simulink model "torpedo"  (Simulink 7.6)
settings: Solver=FixedStepDiscrete  StartTime=0.0  StopTime=0  FixedStep=1/30  RelTol=1e-3
values from neighbouring files (symbols this model uses):
  Forward_Camera_Dimensions = [640 480]    [VisionConstants.m]
  Iter_Segment_Thresh = 60    [VisionConstants.m]
undefined symbols (not defined in the file or in its folder): a_range, b_range, eccent_range, extent_range, Rec, SDTV
libraries: vipgeotforms x3, vipconversions x1
settings Model: Creator=auvt  LastModifiedBy=auvt
settings RTWCC: TargetLang=C++

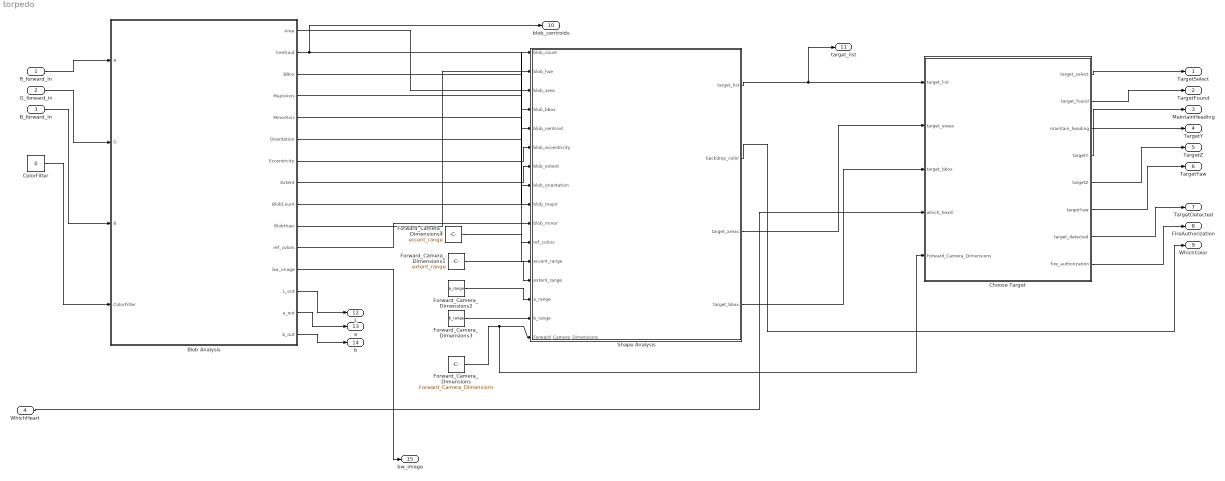
== system torpedo ==
  R_forward_in : Inport  PortDimensions=Forward_Camera_Dimensions
  G_forward_in : Inport  Port=2  PortDimensions=Forward_Camera_Dimensions
  B_forward_in : Inport  Port=3  PortDimensions=Forward_Camera_Dimensions
  WhichHeart : Inport  Port=4
  Blob Analysis : Subsystem
  Choose Target : Stateflow chart  TreatAsAtomicUnit=on
  ColorFilter : Constant  Value=0  SampleTime=-1
  Forward_Camera_Dimensions : Constant  Value=Forward_Camera_Dimensions  SampleTime=-1
  Forward_Camera_Dimensions1 : Constant  Value=extent_range  SampleTime=-1
  Forward_Camera_Dimensions2 : Constant  Value=a_range  SampleTime=-1
  Forward_Camera_Dimensions3 : Constant  Value=b_range  SampleTime=-1
  Forward_Camera_Dimensions4 : Constant  Value=eccent_range  SampleTime=-1
  Shape Analysis : Stateflow chart  TreatAsAtomicUnit=on
  TargetSelect : Outport  OutDataTypeStr=double
  TargetFound : Outport  Port=2  OutDataTypeStr=double
  MaintainHeading : Outport  Port=3  OutDataTypeStr=double
  TargetY : Outport  Port=4  OutDataTypeStr=double
  TargetZ : Outport  Port=5  OutDataTypeStr=double
  TargetYaw : Outport  Port=6  OutDataTypeStr=double
  TargetDetected : Outport  Port=7  OutDataTypeStr=double
  FireAuthorization : Outport  Port=8  OutDataTypeStr=double
  WhichColor : Outport  Port=9  OutDataTypeStr=double
  blob_centroids : Outport  Port=10  OutDataTypeStr=double
  target_list : Outport  Port=11  OutDataTypeStr=double
  L : Outport  Port=12
  a : Outport  Port=13
  b : Outport  Port=14
  bw_image : Outport  Port=15  OutDataTypeStr=double
  wires:
  Shape Analysis/2(backdrop_color) -> WhichColor/1
  Shape Analysis/1(target_list) -> Choose Target/1(target_list), target_list/1
  WhichHeart/1 -> Choose Target/4(which_heart)
  Choose Target/1(target_select) -> TargetSelect/1
  Choose Target/2(target_found) -> TargetFound/1
  Choose Target/3(maintain_heading) -> MaintainHeading/1
  Choose Target/4(targetY) -> TargetY/1
  Choose Target/5(targetZ) -> TargetZ/1
  Choose Target/6(targetYaw) -> TargetYaw/1
  Choose Target/7(target_detected) -> TargetDetected/1
  Choose Target/8(fire_authorization) -> FireAuthorization/1
  Shape Analysis/3(target_areas) -> Choose Target/2(target_areas)
  Shape Analysis/4(target_bbox) -> Choose Target/3(target_bbox)
  Forward_Camera_Dimensions/1 -> Shape Analysis/16(Forward_Camera_Dimensions), Choose Target/5(Forward_Camera_Dimensions)
  Forward_Camera_Dimensions3/1 -> Shape Analysis/15(b_range)
  Forward_Camera_Dimensions2/1 -> Shape Analysis/14(a_range)
  Forward_Camera_Dimensions1/1 -> Shape Analysis/13(extent_range)
  Forward_Camera_Dimensions4/1 -> Shape Analysis/12(eccent_range)
  R_forward_in/1 -> Blob Analysis/1(R)
  G_forward_in/1 -> Blob Analysis/2(G)
  B_forward_in/1 -> Blob Analysis/3(B)
  ColorFilter/1 -> Blob Analysis/4(ColorFilter)
  Blob Analysis/1(Area) -> Shape Analysis/3(blob_area)
  Blob Analysis/9(BlobCount) -> Shape Analysis/1(blob_count)
  Blob Analysis/10(BlobHues) -> Shape Analysis/2(blob_hue)
  Blob Analysis/3(BBox) -> Shape Analysis/4(blob_bbox)
  Blob Analysis/2(Centroid) -> Shape Analysis/5(blob_centroid), blob_centroids/1
  Blob Analysis/7(Eccentricity) -> Shape Analysis/6(blob_eccentricity)
  Blob Analysis/8(Extent) -> Shape Analysis/7(blob_extent)
  Blob Analysis/6(Orientation) -> Shape Analysis/8(blob_orientation)
  Blob Analysis/4(MajorAxis) -> Shape Analysis/9(blob_major)
  Blob Analysis/5(MinorAxis) -> Shape Analysis/10(blob_minor)
  Blob Analysis/11(ref_colors) -> Shape Analysis/11(ref_colors)
  Blob Analysis/13(L_out) -> L/1
  Blob Analysis/14(a_out) -> a/1
  Blob Analysis/15(b_out) -> b/1
  Blob Analysis/12(bw_image) -> bw_image/1

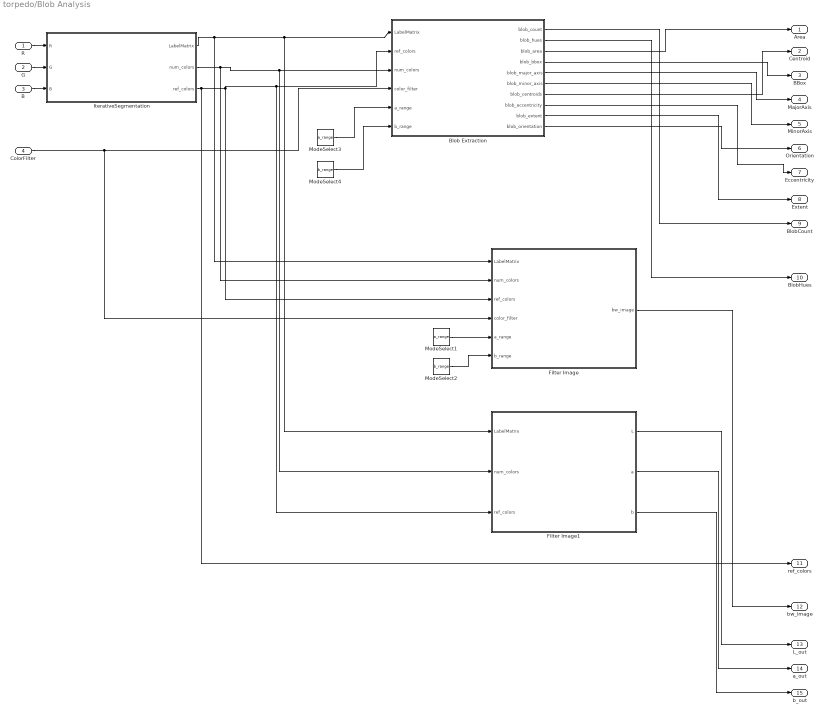
== system torpedo/Blob Analysis ==
  R : Inport
  G : Inport  Port=2
  B : Inport  Port=3
  ColorFilter : Inport  Port=4
  Blob Extraction : Stateflow chart  TreatAsAtomicUnit=on
  Filter Image : Stateflow chart  TreatAsAtomicUnit=on
  Filter Image1 : Stateflow chart  TreatAsAtomicUnit=on
  IterativeSegmentation : Subsystem
      settings: UndoDeleteFcn=Stateflow.SLINSF.SimulinkMan.restorePreDeleteFcn  PreDeleteFcn=Stateflow.SLINSF.SimulinkMan.removePreDeleteFcn
  ModeSelect1 : Constant  Value=a_range  SampleTime=-1
  ModeSelect2 : Constant  Value=b_range  SampleTime=-1
  ModeSelect3 : Constant  Value=a_range  SampleTime=-1
  ModeSelect4 : Constant  Value=b_range  SampleTime=-1
  Area : Outport
  Centroid : Outport  Port=2
  BBox : Outport  Port=3
  MajorAxis : Outport  Port=4
  MinorAxis : Outport  Port=5
  Orientation : Outport  Port=6
  Eccentricity : Outport  Port=7
  Extent : Outport  Port=8
  BlobCount : Outport  Port=9
  BlobHues : Outport  Port=10
  ref_colors : Outport  Port=11
  bw_image : Outport  Port=12
  L_out : Outport  Port=13
  a_out : Outport  Port=14
  b_out : Outport  Port=15
  wires:
  R/1 -> IterativeSegmentation/1(R)
  G/1 -> IterativeSegmentation/2(G)
  B/1 -> IterativeSegmentation/3(B)
  IterativeSegmentation/1(LabelMatrix) -> Filter Image/1(LabelMatrix), Blob Extraction/1(LabelMatrix), Filter Image1/1(LabelMatrix)
  IterativeSegmentation/2(num_colors) -> Filter Image/2(num_colors), Blob Extraction/3(num_colors), Filter Image1/2(num_colors)
  IterativeSegmentation/3(ref_colors) -> Filter Image/3(ref_colors), Blob Extraction/2(ref_colors), Filter Image1/3(ref_colors), ref_colors/1
  ModeSelect1/1 -> Filter Image/5(a_range)
  ModeSelect2/1 -> Filter Image/6(b_range)
  ModeSelect3/1 -> Blob Extraction/5(a_range)
  ModeSelect4/1 -> Blob Extraction/6(b_range)
  ColorFilter/1 -> Blob Extraction/4(color_filter), Filter Image/4(color_filter)
  Blob Extraction/3(blob_area) -> Area/1
  Blob Extraction/7(blob_centroids) -> Centroid/1
  Blob Extraction/4(blob_bbox) -> BBox/1
  Blob Extraction/5(blob_major_axis) -> MajorAxis/1
  Blob Extraction/6(blob_minor_axis) -> MinorAxis/1
  Blob Extraction/10(blob_orientation) -> Orientation/1
  Blob Extraction/8(blob_eccentricity) -> Eccentricity/1
  Blob Extraction/9(blob_extent) -> Extent/1
  Blob Extraction/1(blob_count) -> BlobCount/1
  Blob Extraction/2(blob_hues) -> BlobHues/1
  Filter Image/1(bw_image) -> bw_image/1
  Filter Image1/1(L) -> L_out/1
  Filter Image1/2(a) -> a_out/1
  Filter Image1/3(b) -> b_out/1

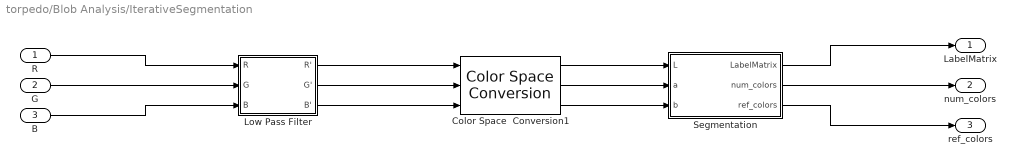
== system torpedo/Blob Analysis/IterativeSegmentation ==
  R : Inport
  G : Inport  Port=2
  B : Inport  Port=3
  Color Space  Conversion1 : vipconversions/Color Space  Conversion  conversion=Obsolete  conversionActive=sR'G'B' to L*a*b*  wp_str=D50  rec=Rec. 601 (SDTV)  sys=1125/60/2:1  imagePorts=Separate color signals
  Low Pass Filter : Subsystem
  Segmentation : Subsystem
  LabelMatrix : Outport
  num_colors : Outport  Port=2
  ref_colors : Outport  Port=3
  wires:
  Segmentation/3(ref_colors) -> ref_colors/1
  Segmentation/2(num_colors) -> num_colors/1
  Segmentation/1(LabelMatrix) -> LabelMatrix/1
  Low Pass Filter/3(B') -> Color Space  Conversion1/3
  Low Pass Filter/2(G') -> Color Space  Conversion1/2
  Low Pass Filter/1(R') -> Color Space  Conversion1/1
  Color Space  Conversion1/3 -> Segmentation/3(b)
  Color Space  Conversion1/2 -> Segmentation/2(a)
  Color Space  Conversion1/1 -> Segmentation/1(L)
  R/1 -> Low Pass Filter/1(R)
  G/1 -> Low Pass Filter/2(G)
  B/1 -> Low Pass Filter/3(B)

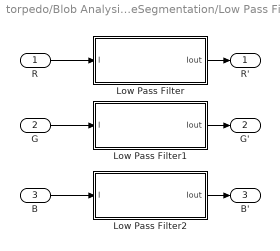
== system torpedo/Blob Analysis/IterativeSegmentation/Low Pass Filter ==
  R : Inport
  G : Inport  Port=2
  B : Inport  Port=3
  Low Pass Filter : Stateflow chart  TreatAsAtomicUnit=on
  Low Pass Filter1 : Stateflow chart  TreatAsAtomicUnit=on
  Low Pass Filter2 : Stateflow chart  TreatAsAtomicUnit=on
  R' : Outport
  G' : Outport  Port=2
  B' : Outport  Port=3
  wires:
  Low Pass Filter/1(Iout) -> R'/1
  Low Pass Filter2/1(Iout) -> B'/1
  Low Pass Filter1/1(Iout) -> G'/1
  B/1 -> Low Pass Filter2/1(I)
  G/1 -> Low Pass Filter1/1(I)
  R/1 -> Low Pass Filter/1(I)

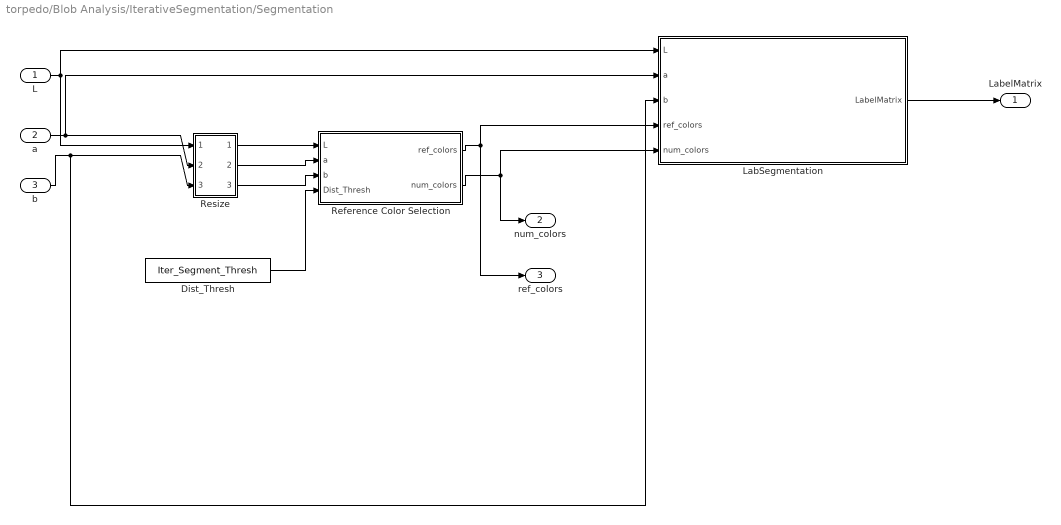
== system torpedo/Blob Analysis/IterativeSegmentation/Segmentation ==
  L : Inport
  a : Inport  Port=2
  b : Inport  Port=3
  Dist_Thresh : Constant  Value=Iter_Segment_Thresh  SampleTime=-1
  LabSegmentation : Stateflow chart  TreatAsAtomicUnit=on
  Reference Color Selection : Stateflow chart  TreatAsAtomicUnit=on
  Resize : Subsystem
  LabelMatrix : Outport
  num_colors : Outport  Port=2
  ref_colors : Outport  Port=3
  wires:
  Dist_Thresh/1 -> Reference Color Selection/4(Dist_Thresh)
  LabSegmentation/1(LabelMatrix) -> LabelMatrix/1
  Reference Color Selection/2(num_colors) -> LabSegmentation/5(num_colors), num_colors/1
  Reference Color Selection/1(ref_colors) -> ref_colors/1, LabSegmentation/4(ref_colors)
  Resize/3(Out3) -> Reference Color Selection/3(b)
  Resize/2(Out2) -> Reference Color Selection/2(a)
  Resize/1(Out1) -> Reference Color Selection/1(L)
  b/1 -> LabSegmentation/3(b), Resize/3(In3)
  a/1 -> LabSegmentation/2(a), Resize/2(In2)
  L/1 -> LabSegmentation/1(L), Resize/1(In1)

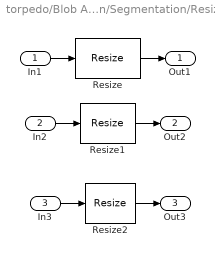
== system torpedo/Blob Analysis/IterativeSegmentation/Segmentation/Resize ==
  In1 : Inport
  In2 : Inport  Port=2
  In3 : Inport  Port=3
  Resize : vipgeotforms/Resize  DialogController=vipDDGCreate  DialogControllerArgs=DataTag0  specify=Number of output rows and columns  rfactor=[]  outCols=25  outRows=25  outRowsCols=[60 80]  interp_method=Bilinear  antialias=on  useROI=off  roiFlag=off  prodOutputMode=Binary point scaling  prodOutputWordLength=32  prodOutputFracLength=10  roundingMode=Nearest  overflowMode=on
  Resize1 : vipgeotforms/Resize  DialogController=vipDDGCreate  DialogControllerArgs=DataTag1  specify=Number of output rows and columns  rfactor=[200 150]  outCols=25  outRows=25  outRowsCols=[60 80]  interp_method=Bilinear  antialias=on  useROI=off  roiFlag=off  prodOutputMode=Binary point scaling  prodOutputWordLength=32  prodOutputFracLength=10  roundingMode=Nearest  overflowMode=on
  Resize2 : vipgeotforms/Resize  DialogController=vipDDGCreate  DialogControllerArgs=DataTag2  specify=Number of output rows and columns  rfactor=[200 150]  outCols=25  outRows=25  outRowsCols=[60 80]  interp_method=Bilinear  antialias=on  useROI=off  roiFlag=off  prodOutputMode=Binary point scaling  prodOutputWordLength=32  prodOutputFracLength=10  roundingMode=Nearest  overflowMode=on
  Out1 : Outport
  Out2 : Outport  Port=2
  Out3 : Outport  Port=3
  wires:
  Resize2/1 -> Out3/1
  In3/1 -> Resize2/1
  Resize1/1 -> Out2/1
  In2/1 -> Resize1/1
  Resize/1 -> Out1/1
  In1/1 -> Resize/1

== matlab function Blob Analysis/Blob Extraction ==
  data: LabelMatrix input double; ref_colors input double; num_colors input double; color_filter input double; blob_count output double; blob_hues output double; blob_area output double; blob_bbox output double; blob_major_axis output double; blob_minor_axis output double; blob_centroids output double; blob_eccentricity output double; blob_extent output double; blob_orientation output double; a_range input double; b_range input double
function [blob_count, blob_hues, blob_area, blob_bbox, blob_major_axis, blob_minor_axis, blob_centroids, blob_eccentricity, blob_extent, blob_orientation] = GetBlobInfo(LabelMatrix, ref_colors, num_colors, color_filter, a_range, b_range)

% This function extracts 
% Input
%   

% Initialize
max_num_blobs = 50;
min_blob_area = 5;

[rows, cols] = size(LabelMatrix);
LogicMatrix = false(rows,cols);

blob_count = 0;
blob_hues = zeros(3,max_num_blobs);

blob_area = -1.*ones(1,max_num_blobs);
blob_bbox = zeros(4,max_num_blobs);
blob_major_axis = zeros(1,max_num_blobs);
blob_minor_axis = zeros(1,max_num_blobs);
blob_centroids = zeros(2,max_num_blobs);
blob_eccentricity = zeros(1,max_num_blobs);
blob_extent = zeros(1,max_num_blobs);
blob_orientation = zeros(1,max_num_blobs);


% Input hblob, a matrix containing [Area, blob_centroids, Eccentricity] for each
% identified blob
persistent hblob
if isempty(hblob)
    hblob = video.BlobAnalysis('AreaOutputPort',true,'CentroidOutputPort',true,...
        'BoundingBoxOutputPort',true,'MajorAxisLengthOutputPort',true,'MinorAxisLengthOutputPort',true,...
        'OrientationOutputPort',true,...
        'EccentricityOutputPort',true,'ExtentOutputPort',true,'NumBlobsOutputPort',true,...
        'MinimumBlobAreaSource','Property','MinimumBlobArea', min_blob_area);
end


% Calculate geometric information about the blobs
%
% LogicMatrix is a binary version of LabelMatrix, with ones at all
%   locations for which color values are k, and zeros everywhere else
for k = 1:num_colors

    a = ref_colors(k, 2);
    b = ref_colors(k, 3);

    if( color_filter == 0 )
        condition = 1;
    else
        if( a >= a_range(1,5) && a <= a_range(2,5) && b >= b_range(1,5) && b <= b_range(2,5) )
            condition = 1;
        else
            condition = 0;
        end
    end
    
    if( condition == 1 )
        
        for i = 1:rows
            for j = 1:cols
                if(LabelMatrix(i,j) ~= k)
                    LogicMatrix(i,j) = false;
                else
                    LogicMatrix(i,j) = true;
                end
            end
        end

        [TArea,TCentroid,TBBox,TMajorAxis,TMinorAxis,TOrientation,TEccent,TExtent,TNumBlobs] = step(hblob,LogicMatrix);

        for i = 1:TNumBlobs
            if(blob_count + TNumBlobs <= max_num_blobs)

                blob_centroids(1,blob_count+i) = TCentroid(1,i);
                blob_centroids(2,blob_count+i) = TCentroid(2,i);

                ii = round(blob_centroids(1,blob_count+i));
                jj = round(blob_centroids(2,blob_count+i));

                blob_hues(1,blob_count+i) = ref_colors( LabelMatrix(ii,jj), 1 );
                blob_hues(2,blob_count+i) = ref_colors( LabelMatrix(ii,jj), 2 );
                blob_hues(3,blob_count+i) = ref_colors( LabelMatrix(ii,jj), 3 );

                blob_area(blob_count+i) = TArea(i);
                blob_bbox(blob_count+i) = TBBox(i);
                blob_major_axis(blob_count+i) = TMajorAxis(i);
                blob_minor_axis(blob_count+i) = TMinorAxis(i);
                blob_eccentricity(blob_count+i) = TEccent(i);
                blob_extent(blob_count+i) = TExtent(i);
                blob_orientation(blob_count+i) = TOrientation(i);

            end
        end

        blob_count = blob_count + double(TNumBlobs);

    end
    
end


return

== matlab function Blob Analysis/Filter Image ==
  data: LabelMatrix input double; num_colors input double; ref_colors input double; color_filter input double; bw_image output double; a_range input double; b_range input double
function bw_image = Filter_Image(LabelMatrix, num_colors, ref_colors, color_filter, a_range, b_range)


% Initialize
[rows,cols] = size(LabelMatrix);
bw_image = zeros(rows,cols);


if( color_filter == 1 )
    
    % Allow only colors in specified range
    for r = 1:rows
        for c = 1:cols

            a = ref_colors(LabelMatrix(r,c), 2);
            b = ref_colors(LabelMatrix(r,c), 3);

            if( a >= a_range(1,5) && a <= a_range(2,5) && b >= b_range(1,5) && b <= b_range(2,5) )
                bw_image(r,c) = 1;
            end

        end
    end
    
else
    
    % Generate a bw image using color indices
    maxValue = max(max(max(LabelMatrix)));
    if(maxValue == 0)
        maxValue = 1;
    end
    for r = 1:rows
        for c = 1:cols
            bw_image(r,c) = LabelMatrix(r,c)/maxValue;
        end
    end
    
end


return

== matlab function Blob Analysis/Filter Image1 ==
  data: LabelMatrix input double; num_colors input double; ref_colors input double; L output double; a output double; b output double
function [L, a, b] = Display_Image(LabelMatrix, num_colors, ref_colors)


% Initialize
[rows,cols] = size(LabelMatrix);
bw_image = zeros(rows,cols);
L = zeros(rows,cols);
a = zeros(rows,cols);
b = zeros(rows,cols);


% Allow only colors in specified range
for r = 1:rows
    for c = 1:cols
        
        L(r,c) = ref_colors(LabelMatrix(r,c), 1);
        a(r,c) = ref_colors(LabelMatrix(r,c), 2);
        b(r,c) = ref_colors(LabelMatrix(r,c), 3);
        
    end
end


return

== matlab function Blob Analysis/IterativeSegmentation/Low Pass Filter/Low Pass Filter ==
  data: I input double; Iout output double
function Iout = GaussianBlurr(I)
% This function calculates the gaussian blur of an intensity image

sigma = sqrt(2);

Grows = 3;    % Gaussian matrix rows
Gcols = 3;    % Gaussian matrix columns

[Irows Icols] = size(I);

Iout = double(zeros(Irows,Icols));

Trows = Irows - Grows + 1;
Tcols = Icols - Gcols + 1;
Itemp = double(zeros(Trows,Tcols));

G = zeros(Grows,Gcols);

FirstRow = ceil(-Grows/2);
LastRow = floor(Grows/2);
FirstCol = ceil(-Gcols/2);
LastCol = floor(Gcols/2);
Gsum = 0;
for i=FirstRow:LastRow
    for j = FirstCol:LastCol
        G(i-FirstRow+1,j-FirstCol+1) = exp(-(j*j+i*i)/(2*sigma*sigma));
        Gsum = Gsum + G(i-FirstRow+1,j-FirstCol+1);
    end
end

G = G./Gsum;

Itemp = conv2(double(I),double(G),'valid');

% reflect boundaries to keep image the same size
% top
Iout((1:LastRow),(LastCol+1:Icols-LastCol)) = Itemp((1:LastRow),(1:Tcols));
% bottom
Iout((Irows-LastRow+1:Irows),(LastCol+1:Icols-LastCol)) = Itemp((Trows-LastRow+1:Trows),(1:Tcols));
% left
Iout((1+LastRow:Irows-LastRow),(1:LastCol)) = Itemp((1:Trows),(1:LastCol));
% right
Iout((1+LastRow:Irows-LastRow),(Icols-LastCol+1:Icols)) = Itemp((1:Trows),(Tcols-LastCol+1:Tcols));
% center
Iout((1+LastRow:Irows-LastRow),(1+LastCol:Icols-LastCol)) = Itemp;
% top left corner
Iout(1:LastRow,1:LastCol) = Itemp(1:LastRow,1:LastCol);
% top right corner
Iout(1:LastRow,Icols-LastCol:Icols) = Itemp(1:LastRow,Tcols-LastCol:Tcols);
% bottom left corner
Iout(Irows-LastRow:Irows,1:LastCol) = Itemp(Trows-LastRow:Trows,1:LastCol);
% bottom right corner
Iout(Irows-LastRow:Irows,Icols-LastCol:Icols) = Itemp(Trows-LastRow:Trows,Tcols-LastCol:Tcols);

return

== matlab function Blob Analysis/IterativeSegmentation/Low Pass Filter/Low Pass Filter1 ==
  data: I input double; Iout output double
function Iout = GaussianBlurr(I)
% This function calculates the gaussian blur of an intensity image

sigma = sqrt(2);

Grows = 3;    % Gaussian matrix rows
Gcols = 3;    % Gaussian matrix columns

[Irows Icols] = size(I);

Iout = double(zeros(Irows,Icols));

Trows = Irows - Grows + 1;
Tcols = Icols - Gcols + 1;
Itemp = double(zeros(Trows,Tcols));

G = zeros(Grows,Gcols);

FirstRow = ceil(-Grows/2);
LastRow = floor(Grows/2);
FirstCol = ceil(-Gcols/2);
LastCol = floor(Gcols/2);
Gsum = 0;
for i=FirstRow:LastRow
    for j = FirstCol:LastCol
        G(i-FirstRow+1,j-FirstCol+1) = exp(-(j*j+i*i)/(2*sigma*sigma));
        Gsum = Gsum + G(i-FirstRow+1,j-FirstCol+1);
    end
end

G = G./Gsum;

Itemp = conv2(double(I),double(G),'valid');

% reflect boundaries to keep image the same size
% top
Iout((1:LastRow),(LastCol+1:Icols-LastCol)) = Itemp((1:LastRow),(1:Tcols));
% bottom
Iout((Irows-LastRow+1:Irows),(LastCol+1:Icols-LastCol)) = Itemp((Trows-LastRow+1:Trows),(1:Tcols));
% left
Iout((1+LastRow:Irows-LastRow),(1:LastCol)) = Itemp((1:Trows),(1:LastCol));
% right
Iout((1+LastRow:Irows-LastRow),(Icols-LastCol+1:Icols)) = Itemp((1:Trows),(Tcols-LastCol+1:Tcols));
% center
Iout((1+LastRow:Irows-LastRow),(1+LastCol:Icols-LastCol)) = Itemp;
% top left corner
Iout(1:LastRow,1:LastCol) = Itemp(1:LastRow,1:LastCol);
% top right corner
Iout(1:LastRow,Icols-LastCol:Icols) = Itemp(1:LastRow,Tcols-LastCol:Tcols);
% bottom left corner
Iout(Irows-LastRow:Irows,1:LastCol) = Itemp(Trows-LastRow:Trows,1:LastCol);
% bottom right corner
Iout(Irows-LastRow:Irows,Icols-LastCol:Icols) = Itemp(Trows-LastRow:Trows,Tcols-LastCol:Tcols);

return

== matlab function Blob Analysis/IterativeSegmentation/Low Pass Filter/Low Pass Filter2 ==
  data: I input double; Iout output double
function Iout = GaussianBlurr(I)
% This function calculates the gaussian blur of an intensity image

sigma = sqrt(2);

Grows = 3;    % Gaussian matrix rows
Gcols = 3;    % Gaussian matrix columns

[Irows Icols] = size(I);

Iout = double(zeros(Irows,Icols));

Trows = Irows - Grows + 1;
Tcols = Icols - Gcols + 1;
Itemp = double(zeros(Trows,Tcols));

G = zeros(Grows,Gcols);

FirstRow = ceil(-Grows/2);
LastRow = floor(Grows/2);
FirstCol = ceil(-Gcols/2);
LastCol = floor(Gcols/2);
Gsum = 0;
for i=FirstRow:LastRow
    for j = FirstCol:LastCol
        G(i-FirstRow+1,j-FirstCol+1) = exp(-(j*j+i*i)/(2*sigma*sigma));
        Gsum = Gsum + G(i-FirstRow+1,j-FirstCol+1);
    end
end

G = G./Gsum;

Itemp = conv2(double(I),double(G),'valid');

% reflect boundaries to keep image the same size
% top
Iout((1:LastRow),(LastCol+1:Icols-LastCol)) = Itemp((1:LastRow),(1:Tcols));
% bottom
Iout((Irows-LastRow+1:Irows),(LastCol+1:Icols-LastCol)) = Itemp((Trows-LastRow+1:Trows),(1:Tcols));
% left
Iout((1+LastRow:Irows-LastRow),(1:LastCol)) = Itemp((1:Trows),(1:LastCol));
% right
Iout((1+LastRow:Irows-LastRow),(Icols-LastCol+1:Icols)) = Itemp((1:Trows),(Tcols-LastCol+1:Tcols));
% center
Iout((1+LastRow:Irows-LastRow),(1+LastCol:Icols-LastCol)) = Itemp;
% top left corner
Iout(1:LastRow,1:LastCol) = Itemp(1:LastRow,1:LastCol);
% top right corner
Iout(1:LastRow,Icols-LastCol:Icols) = Itemp(1:LastRow,Tcols-LastCol:Tcols);
% bottom left corner
Iout(Irows-LastRow:Irows,1:LastCol) = Itemp(Trows-LastRow:Trows,1:LastCol);
% bottom right corner
Iout(Irows-LastRow:Irows,Icols-LastCol:Icols) = Itemp(Trows-LastRow:Trows,Tcols-LastCol:Tcols);

return

== matlab function Blob Analysis/IterativeSegmentation/Segmentation/LabSegmentation ==
  data: L input double; LabelMatrix output double; a input double; b input double; ref_colors input double; num_colors input double
function LabelMatrix  = LabSegmentation(L,a,b,ref_colors,num_colors)
% This function generates the label matrix

[rows cols] = size(L);

Lout = zeros(rows,cols);
aout = zeros(rows,cols);
bout = zeros(rows,cols);

LabelMatrix = zeros(rows,cols);

for i = 1:rows
    for j = 1:cols
        min_dist = 1000;
        index = 1;
        for k = 1:num_colors
            dist = sqrt((ref_colors(k,1) - L(i,j))^2 + (ref_colors(k,2) - a(i,j))^2 + (ref_colors(k,3) - b(i,j))^2);
            if(dist < min_dist)
                min_dist = double(dist);
                index = k;
            end
        end
        LabelMatrix(i,j) = index;
    end
end

for i = 1:rows
    for j = 1:cols
        Lout(i,j) = ref_colors(LabelMatrix(i,j),1);
        aout(i,j) = ref_colors(LabelMatrix(i,j),2);
        bout(i,j) = ref_colors(LabelMatrix(i,j),3);
    end
end

cow = 1;

return

== matlab function Blob Analysis/IterativeSegmentation/Segmentation/Reference Color Selection ==
  data: L input double; ref_colors output double; a input double; b input double; num_colors output double; Dist_Thresh input double
function [ref_colors, num_colors] = Segmentation(L,a,b,Dist_Thresh)
% This function tries segmentation by adding new reference colors everytime
% a pixel is found with a distance greater than a certain amount from
% every other reference color

[rows cols] = size(L);

Dist_Threshold = Dist_Thresh;% L = 0 to 100, a = -100 to 100, b = -100 to 100
                    % max dist = 300 -> 60/300 is 20%
x = 1;  % coefficients determining distance calculation
y = 1.5;
z = 1.5;

max_num_colors = 50;
ref_colors = zeros(max_num_colors,3);   % At most 50 different reference colors
LabelMatrix = zeros(rows,cols);
num_colors = 1;

center_row = floor(rows/2);
center_col = floor(cols/2);

% Define first reference color to be colr
ref_colors(1,:) = [L(center_row,center_col) a(center_row,center_col) b(center_row,center_col)];

flag = 0;
i = 1;
j = 1;
while(i <= rows)        % perform initial segmentation
    while(i <= rows && flag == 0)
        while(j <= cols && flag == 0)
            k = 1;
            min_dist = 1000;
            index = 1;
            while(k <= num_colors)
                dist = sqrt(x*(ref_colors(k,1) - L(i,j))^2 + y*(ref_colors(k,2) - a(i,j))^2 + z*(ref_colors(k,3) - b(i,j))^2);
                if(min_dist > dist)
                    min_dist = double(dist);
                    index = k;
                end
                k = k + 1;
            end
            if(j == 117)
                cow = 1;
            end
            if(min_dist > Dist_Threshold && num_colors < max_num_colors)
                ref_colors(num_colors+1,:) = [L(i,j) a(i,j) b(i,j)];
                num_colors = num_colors + 1;
                flag = 1;
                i = 0;
                j = 0;
            else
                LabelMatrix(i,j) = index;
            end
            j = j + 1;
        end
        j = 1;
        i = i + 1;
    end
    flag = 0;
end

% Go through image once more to get more accurate values for the different regions
ref_color_L_avg = zeros(50,1);
ref_color_a_avg = zeros(50,1);
ref_color_b_avg = zeros(50,1);
color_count = zeros(50,1);
for i = 1:rows
    for j = 1:cols
        index = LabelMatrix(i,j);
        ref_color_L_avg(index) = ref_color_L_avg(index) + L(i,j);
        ref_color_a_avg(index) = ref_color_a_avg(index) + a(i,j);
        ref_color_b_avg(index) = ref_color_b_avg(index) + b(i,j);
        color_count(index) = color_count(index) + 1;
    end
end
ref_color_L_avg = ref_color_L_avg ./ color_count;
ref_color_a_avg = ref_color_a_avg ./ color_count;
ref_color_b_avg = ref_color_b_avg ./ color_count;

for i = 1:num_colors
    ref_colors(i,1) = ref_color_L_avg(i);
    ref_colors(i,2) = ref_color_a_avg(i);
    ref_colors(i,3) = ref_color_b_avg(i);
end

return

== matlab function Choose Target ==
  data: target_list input double; target_areas input double; target_bbox input double; which_heart input double; target_select output double; target_found output double; maintain_heading output double; targetY output double; targetZ output double; targetYaw output double; target_detected output double; Forward_Camera_Dimensions input double; fire_authorization output double
function [target_select, target_found, maintain_heading, targetY, targetZ, targetYaw, target_detected, fire_authorization] = Choose_Target(target_list, target_areas, target_bbox, which_heart, Forward_Camera_Dimensions)
% This function takes in vectors representing targets present in the image,
%   and decides which heart to target.
%
% Input
%   target_list = 2xN matrix of centroids for identified targets
%                 1st column -> backdrop
%                 2nd column -> large heart
%                 3rd column -> small heart
%   which_heart = which heart target should be targeted
%               = 0 -> Use default
%               = 1 -> Target large heart
%               = 2 -> Target small heart
%
% Output
%   target_select = input to MotionController.mdl, which selects which
%     camera to use
%   target_found = informs MotionController that a target is being tracked
%   maintain_heading = instructs MotionController to strafe xor turn:
%                    = 0 -> Turn toward target (use targetYaw)
%                    = 1 -> Strafe to target (use targetY)
%   targetY, targetZ = position of buoy in absolute coordinates
%   targetYaw = relative, lateral angular displacement of target from
%     straight ahead (in degrees)
%   target_detected = informs the script that the correct target is being
%     tracked


% Initialize
target_select = 1;
target_found = 1;
maintain_heading = 1;
targetY = 0;
targetZ = 0;
targetYaw = 0;
target_detected = 0;
fire_authorization = 0;

rows = Forward_Camera_Dimensions(1);
cols = Forward_Camera_Dimensions(2);
image_area = rows*cols;


% Determine which target to track
if(which_heart == 1)
    t = 2;
elseif(which_heart == 2)
    t = 3;
else
    t = 2;
end


% Convert to vehicle-centered coordinate system
targetY = target_list(2,t) - floor(cols/2);
targetZ = target_list(1,t) - floor(rows/2);
targetYaw = 0;
if( target_found(t) ~= 0 )
    target_detected = 1;
end


% Determine if target is centered
bbox_shrink_ratio = .8;  % Scaling factor applied to bounding box side lengths (makes targeting more precise)
max_horizontal_distance = .5*bbox_shrink_ratio*abs( target_bbox(4,t) - target_bbox(3,t) );
max_vertical_distance = .5*bbox_shrink_ratio*abs( target_bbox(2,t) - target_bbox(1,t) );

if( abs(targetY) <= max_horizontal_distance && abs(targetZ) <= max_vertical_distance )
    fire_authorization = 1;
end


% Determine if target is within firing range
target_area_ratio = .2;
if( target_areas(t) / image_area < target_area_ratio )
    fire_authorization = 0;
end


return

== matlab function Shape Analysis ==
  data: blob_count input double; blob_hue input double; blob_area input double; blob_bbox input double; blob_centroid input double; target_list output double; backdrop_color output double; blob_eccentricity input double; blob_extent input double; blob_orientation input double; blob_major input double; blob_minor input double; ref_colors input double; eccent_range input double; extent_range input double; a_range input double; b_range input double; target_areas output double; target_bbox output double; Forward_Camera_Dimensions input double
function [target_list, backdrop_color, target_areas, target_bbox] = Extract_Targets(blob_count, blob_hue, blob_area, blob_bbox, blob_centroid, blob_eccentricity, blob_extent, blob_orientation, blob_major, blob_minor, ref_colors, eccent_range, extent_range, a_range, b_range, Forward_Camera_Dimensions)
% This function takes in vectors representing blobs present in the image,
%   and returns information about how many and what kind of targets are
%   present. Targets are identified by shape only.
%
% Input
%   blob_count = number of blobs identified
%   blob_hue = 3xN matrix of blob Lab components
%   blob_area = 1xN vector of blob areas
%   blob_bbox = 4xN matrix of blob bounding boxes (r,r,c,c)
%   blob_centroid = 2xN matrix of blob centroids (r,c)
%   blob_eccentricity = 1xN vector of eccentricities
%   blob_extent = 1xN vector of eccentricities
%   blob_orientation = 1xN vector of angle b/n major axis and horizontal
%     axis (radians, positive ccw)
%   blob_major = 1xN vector of major axis lengths
%   blob_minor = 1xN vector of minor axis lengths
%   ref_colors = Nx3 matrix of Lab components from segmentation
%
%   extent_range = 2xN matrix of ranges which distinguish shapes
%                  1st column -> backdrop
%                  2nd column -> heart
%   eccent_range = 2xN matrix of ranges which distinguish shapes
%                  1st column -> backdrop
%                  2nd column -> heart
%   a_range, b_range = 2xN matrix of lower/upper bounds on a, b for each
%     color
%
% Internal
%   target_found = 1xN vector indicating whether or not each target has
%     been identified
%                = 0 -> No target identified
%                = b -> Index in blob vectors corresponding to target
%
% Output
%   target_list = 2xN matrix of centroids for identified targets
%                 1st column -> backdrop
%                 2nd column -> large heart
%                 3rd column -> small heart
%   backdrop_color = color of backdrop
%                  = 0 -> Not identified
%                  = 3 -> Blue
%                  = 4 -> Red
%   target_areas = 1xN vector of target areas
%   target_bbox = 4xN matrix of target bounding boxes


% Initialize
target_found = zeros(1,3);
target_list = zeros(2,3);
backdrop_color = 0;
target_areas = zeros(1,3);
target_bbox = zeros(4,3);

max_num_colors = size(a_range,2);
rows = Forward_Camera_Dimensions(1);
cols = Forward_Camera_Dimensions(2);
image_area = rows*cols;
area_thresh = 0.8;  % Ratio of blob area to image area considered to imply the blob is actually background noise


% Store target information if geometric conditions are met
%   Conditions: 1) Blob eccentricity is within specified range
%               2) Blob extent is within specified range
for b = 1:blob_count
    
    % Backdrop
    if( (blob_area(b)/image_area <= area_thresh) && (blob_extent(b) >= extent_range(1,1)) && (blob_extent(b) <= extent_range(2,1)) && (blob_eccentricity(b) >= eccent_range(1,1)) && (blob_eccentricity(b) <= eccent_range(2,1)) )
        
        % Check that a bigger backdrop has not already been identified
        if(target_found(1) ~= 0)
            if(blob_area(b) > blob_area(target_found(1)))
                target_found(1) = b;
            end
        else
            target_found(1) = b;
        end
        
    end
    
    % Heart
    if( (blob_extent(b) >= extent_range(1,2)) && (blob_extent(b) <= extent_range(2,2)) && (blob_eccentricity(b) >= eccent_range(1,2)) && (blob_eccentricity(b) <= eccent_range(2,2)) )
        
        % Target the blob if it has a valid range
        if(target_found(2) == 0)
            target_found(2) = b;
        elseif(target_found(3) == 0)
            target_found(3) = b;
        end
        
    end
    
end


% Swap heart targets as needed so the target order in target_list is
%   [backdrop, large heart, small heart]
swap_var = target_found(2);
if( target_found(2) ~= 0 && target_found(3) ~= 0 )
    if( blob_area(target_found(2)) < blob_area(target_found(3)) )
        target_found(2) = target_found(3);
        target_found(3) = swap_var;
    end
end


% Store target centroids and areas
for t = 1:3
    tf = target_found(t);
    if( tf ~= 0 )
        target_list(1,t) = blob_centroid(1,tf);
        target_list(2,t) = blob_centroid(2,tf);
        target_areas(t) = blob_area(tf);
        target_bbox(1,t) = blob_bbox(1,tf);
        target_bbox(2,t) = blob_bbox(2,tf);
        target_bbox(3,t) = blob_bbox(3,tf);
        target_bbox(4,t) = blob_bbox(4,tf);
    end
end


% Determine backdrop color according to a_range and b_range
if( target_found(1) ~= 0 )
    a = blob_hue(2,target_found(1));
    b = blob_hue(3,target_found(1));
    for col = 1:max_num_colors
        if( a >= a_range(1,col) && a <= a_range(2,col) && b >= b_range(1,col) && b <= b_range(2,col) )
            backdrop_color = col;
            break;
        end
    end
end


% Correct any mis-identified colors
if( (backdrop_color ~= 0) && (backdrop_color ~= 3) && (backdrop_color ~= 3) )
    
    if(backdrop_color == 0)
        backdrop_color = 4;
    elseif(backdrop_color == 1)
        backdrop_color = 3;
    elseif(backdrop_color == 2)
        backdrop_color = 3;
    elseif(backdrop_color == 5)
        backdrop_color = 4;
    elseif(backdrop_color == 6)
        backdrop_color = 4;
    elseif(backdrop_color == 7)
        backdrop_color = 3;
    else
        backdrop_color = 0;
    end
    
end


return
